simulink model "pipelined_and_spatial_parallelism"  (R2015b)
settings: Solver=FixedStepDiscrete  SolverMode=SingleTasking  StartTime=0.0  StopTime=5e-4  RelTol=1e-3
undefined symbols (not defined in the file): a, b
libraries: shlslibv1 x5277
(part 3 of 23)

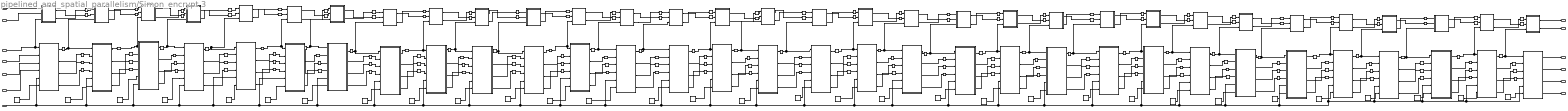
== system pipelined_and_spatial_parallelism/Simon_encrypt 3 ==
  x_i1 : Inport
  x_i : Inport  Port=2
  k_i : Inport  Port=3
  k_i1 : Inport  Port=4
  k_i2 : Inport  Port=5
  k_i3 : Inport  Port=6
  c : Inport  Port=7
  Delay{1..186} (186 alike) : shlslibv1/Memories/Delay  syn_delay_val=1  synBlockType=primitive  synLatency=1  synBlockId=104
  Key_expansion_function : Subsystem
  Key_expansion_function1 : Subsystem
  Key_expansion_function10 : Subsystem
  Key_expansion_function11 : Subsystem
  Key_expansion_function12 : Subsystem
  Key_expansion_function13 : Subsystem
  Key_expansion_function14 : Subsystem
  Key_expansion_function15 : Subsystem
  Key_expansion_function16 : Subsystem
  Key_expansion_function17 : Subsystem
  Key_expansion_function18 : Subsystem
  Key_expansion_function19 : Subsystem
  Key_expansion_function2 : Subsystem
  Key_expansion_function20 : Subsystem
  Key_expansion_function21 : Subsystem
  Key_expansion_function22 : Subsystem
  Key_expansion_function23 : Subsystem
  Key_expansion_function24 : Subsystem
  Key_expansion_function25 : Subsystem
  Key_expansion_function26 : Subsystem
  Key_expansion_function27 : Subsystem
  Key_expansion_function29 : Subsystem
  Key_expansion_function3 : Subsystem
  Key_expansion_function30 : Subsystem
  Key_expansion_function31 : Subsystem
  Key_expansion_function32 : Subsystem
  Key_expansion_function4 : Subsystem
  Key_expansion_function5 : Subsystem
  Key_expansion_function6 : Subsystem
  Key_expansion_function7 : Subsystem
  Key_expansion_function8 : Subsystem
  Key_expansion_function9 : Subsystem
  Round_function : Subsystem
  Round_function1 : Subsystem
  Round_function10 : Subsystem
  Round_function11 : Subsystem
  Round_function12 : Subsystem
  Round_function13 : Subsystem
  Round_function14 : Subsystem
  Round_function15 : Subsystem
  Round_function16 : Subsystem
  Round_function17 : Subsystem
  Round_function18 : Subsystem
  Round_function19 : Subsystem
  Round_function2 : Subsystem
  Round_function20 : Subsystem
  Round_function21 : Subsystem
  Round_function22 : Subsystem
  Round_function23 : Subsystem
  Round_function24 : Subsystem
  Round_function25 : Subsystem
  Round_function26 : Subsystem
  Round_function27 : Subsystem
  Round_function29 : Subsystem
  Round_function3 : Subsystem
  Round_function30 : Subsystem
  Round_function31 : Subsystem
  Round_function32 : Subsystem
  Round_function4 : Subsystem
  Round_function5 : Subsystem
  Round_function6 : Subsystem
  Round_function7 : Subsystem
  Round_function8 : Subsystem
  Round_function9 : Subsystem
  Sequence{,1..4,6,10,13,15,17..18,23..25,28..29} (16 alike) : shlslibv1/Sources/Sequence  syn_seq_vec=[1]  syn_seq_wl=16  syn_seq_fl=0  syn_seq_dt=unsigned  syn_rst_port=off  syn_en_port=off  syn_seq_st=-1  synBlockType=custom  synLatency=1
  Sequence{5,7..9,11..12,14,16,19..22,26..27,30..31} (16 alike) : shlslibv1/Sources/Sequence  syn_seq_vec=[0]  syn_seq_wl=16  syn_seq_fl=0  syn_seq_dt=unsigned  syn_rst_port=off  syn_en_port=off  syn_seq_st=-1  synBlockType=custom  synLatency=1
  X_iiii : Outport
  X_iiii1 : Outport  Port=2
  K_iiii : Outport  Port=3
  K_iiiii1 : Outport  Port=4
  K_iiii2 : Outport  Port=5
  K_iiii3 : Outport  Port=6
  wires:
  Key_expansion_function/2(Kiii1) -> Delay11/1
  Key_expansion_function/3(Kiii2) -> Delay12/1
  Key_expansion_function/4(Kiii3) -> Delay13/1
  x_i1/1 -> Round_function/1(" x_ii1")
  x_i/1 -> Round_function/2(x_ii)
  k_i/1 -> Round_function/3(k_i), Key_expansion_function/1(k_ii)
  k_i1/1 -> Key_expansion_function/2(k_ii1)
  k_i2/1 -> Key_expansion_function/3(k_ii2)
  k_i3/1 -> Key_expansion_function/4(k_ii3)
  Round_function/2(xiii2) -> Delay7/1
  Round_function/1(Xiii1) -> Delay8/1
  Round_function1/1(Xiii1) -> Delay15/1
  Round_function1/2(xiii2) -> Delay14/1
  Key_expansion_function1/2(Kiii1) -> Delay18/1
  Key_expansion_function1/3(Kiii2) -> Delay19/1
  Key_expansion_function1/4(Kiii3) -> Delay20/1
  Round_function2/1(Xiii1) -> Delay22/1
  Round_function2/2(xiii2) -> Delay21/1
  Key_expansion_function2/2(Kiii1) -> Delay25/1
  Key_expansion_function2/3(Kiii2) -> Delay26/1
  Key_expansion_function2/4(Kiii3) -> Delay27/1
  Delay7/1 -> Round_function1/1(" x_ii1")
  Delay8/1 -> Round_function1/2(x_ii)
  Key_expansion_function/1(K_iii) -> Delay9/1
  Delay11/1 -> Key_expansion_function1/2(k_ii1)
  Delay12/1 -> Key_expansion_function1/3(k_ii2)
  Delay13/1 -> Key_expansion_function1/4(k_ii3)
  Delay14/1 -> Round_function2/1(" x_ii1")
  Delay15/1 -> Round_function2/2(x_ii)
  Key_expansion_function1/1(K_iii) -> Delay10/1
  Delay18/1 -> Key_expansion_function2/2(k_ii1)
  Delay19/1 -> Key_expansion_function2/3(k_ii2)
  Delay20/1 -> Key_expansion_function2/4(k_ii3)
  Delay21/1 -> Round_function3/1(" x_ii1")
  Delay22/1 -> Round_function3/2(x_ii)
  Key_expansion_function2/1(K_iii) -> Delay16/1
  Delay25/1 -> Key_expansion_function3/2(k_ii1)
  Delay26/1 -> Key_expansion_function3/3(k_ii2)
  Delay27/1 -> Key_expansion_function3/4(k_ii3)
  Delay9/1 -> Key_expansion_function1/1(k_ii), Round_function1/3(k_i)
  Delay10/1 -> Round_function2/3(k_i), Key_expansion_function2/1(k_ii)
  Delay16/1 -> Key_expansion_function3/1(k_ii), Round_function3/3(k_i)
  Key_expansion_function3/2(Kiii1) -> Delay2/1
  Key_expansion_function3/3(Kiii2) -> Delay3/1
  Key_expansion_function3/4(Kiii3) -> Delay4/1
  Round_function3/2(xiii2) -> Delay34/1
  Round_function3/1(Xiii1) -> Delay35/1
  Round_function4/1(Xiii1) -> Delay6/1
  Round_function4/2(xiii2) -> Delay5/1
  Key_expansion_function4/2(Kiii1) -> Delay23/1
  Key_expansion_function4/3(Kiii2) -> Delay24/1
  Key_expansion_function4/4(Kiii3) -> Delay28/1
  Round_function5/1(Xiii1) -> Delay30/1
  Round_function5/2(xiii2) -> Delay29/1
  Key_expansion_function5/2(Kiii1) -> Delay31/1
  Key_expansion_function5/3(Kiii2) -> Delay32/1
  Key_expansion_function5/4(Kiii3) -> Delay33/1
  Delay34/1 -> Round_function4/1(" x_ii1")
  Delay35/1 -> Round_function4/2(x_ii)
  Key_expansion_function3/1(K_iii) -> Delay36/1
  Delay2/1 -> Key_expansion_function4/2(k_ii1)
  Delay3/1 -> Key_expansion_function4/3(k_ii2)
  Delay4/1 -> Key_expansion_function4/4(k_ii3)
  Delay5/1 -> Round_function5/1(" x_ii1")
  Delay6/1 -> Round_function5/2(x_ii)
  Key_expansion_function4/1(K_iii) -> Delay1/1
  Delay23/1 -> Key_expansion_function5/2(k_ii1)
  Delay24/1 -> Key_expansion_function5/3(k_ii2)
  Delay28/1 -> Key_expansion_function5/4(k_ii3)
  Delay29/1 -> Round_function6/1(" x_ii1")
  Delay30/1 -> Round_function6/2(x_ii)
  Key_expansion_function5/1(K_iii) -> Delay17/1
  Delay31/1 -> Key_expansion_function6/2(k_ii1)
  Delay32/1 -> Key_expansion_function6/3(k_ii2)
  Delay33/1 -> Key_expansion_function6/4(k_ii3)
  Delay36/1 -> Round_function4/3(k_i), Key_expansion_function4/1(k_ii)
  Delay1/1 -> Key_expansion_function5/1(k_ii), Round_function5/3(k_i)
  Delay17/1 -> Key_expansion_function6/1(k_ii), Round_function6/3(k_i)
  Key_expansion_function6/2(Kiii1) -> Delay39/1
  Key_expansion_function6/3(Kiii2) -> Delay40/1
  Key_expansion_function6/4(Kiii3) -> Delay41/1
  Round_function6/2(xiii2) -> Delay70/1
  Round_function6/1(Xiii1) -> Delay71/1
  Round_function7/1(Xiii1) -> Delay43/1
  Round_function7/2(xiii2) -> Delay42/1
  Key_expansion_function7/2(Kiii1) -> Delay46/1
  Key_expansion_function7/3(Kiii2) -> Delay47/1
  Key_expansion_function7/4(Kiii3) -> Delay49/1
  Round_function8/1(Xiii1) -> Delay51/1
  Round_function8/2(xiii2) -> Delay50/1
  Key_expansion_function8/2(Kiii1) -> Delay54/1
  Key_expansion_function8/3(Kiii2) -> Delay55/1
  Key_expansion_function8/4(Kiii3) -> Delay56/1
  Delay70/1 -> Round_function7/1(" x_ii1")
  Delay71/1 -> Round_function7/2(x_ii)
  Key_expansion_function6/1(K_iii) -> Delay72/1
  Delay39/1 -> Key_expansion_function7/2(k_ii1)
  Delay40/1 -> Key_expansion_function7/3(k_ii2)
  Delay41/1 -> Key_expansion_function7/4(k_ii3)
  Delay42/1 -> Round_function8/1(" x_ii1")
  Delay43/1 -> Round_function8/2(x_ii)
  Key_expansion_function7/1(K_iii) -> Delay38/1
  Delay46/1 -> Key_expansion_function8/2(k_ii1)
  Delay47/1 -> Key_expansion_function8/3(k_ii2)
  Delay49/1 -> Key_expansion_function8/4(k_ii3)
  Delay50/1 -> Round_function9/1(" x_ii1")
  Delay51/1 -> Round_function9/2(x_ii)
  Key_expansion_function8/1(K_iii) -> Delay44/1
  Delay54/1 -> Key_expansion_function9/2(k_ii1)
  Delay55/1 -> Key_expansion_function9/3(k_ii2)
  Delay56/1 -> Key_expansion_function9/4(k_ii3)
  Delay72/1 -> Round_function7/3(k_i), Key_expansion_function7/1(k_ii)
  Delay38/1 -> Round_function8/3(k_i), Key_expansion_function8/1(k_ii)
  Delay44/1 -> Round_function9/3(k_i), Key_expansion_function9/1(k_ii)
  Key_expansion_function9/2(Kiii1) -> Delay48/1
  Key_expansion_function9/3(Kiii2) -> Delay59/1
  Key_expansion_function9/4(Kiii3) -> Delay67/1
  Round_function9/2(xiii2) -> Delay64/1
  Round_function9/1(Xiii1) -> Delay65/1
  Round_function10/1(Xiii1) -> Delay69/1
  Round_function10/2(xiii2) -> Delay68/1
  Key_expansion_function10/2(Kiii1) -> Delay52/1
  Key_expansion_function10/3(Kiii2) -> Delay53/1
  Key_expansion_function10/4(Kiii3) -> Delay57/1
  Round_function11/1(Xiii1) -> Delay60/1
  Round_function11/2(xiii2) -> Delay58/1
  Key_expansion_function11/2(Kiii1) -> Delay61/1
  Key_expansion_function11/3(Kiii2) -> Delay62/1
  Key_expansion_function11/4(Kiii3) -> Delay63/1
  Delay64/1 -> Round_function10/1(" x_ii1")
  Delay65/1 -> Round_function10/2(x_ii)
  Key_expansion_function9/1(K_iii) -> Delay66/1
  Delay48/1 -> Key_expansion_function10/2(k_ii1)
  Delay59/1 -> Key_expansion_function10/3(k_ii2)
  Delay67/1 -> Key_expansion_function10/4(k_ii3)
  Delay68/1 -> Round_function11/1(" x_ii1")
  Delay69/1 -> Round_function11/2(x_ii)
  Key_expansion_function10/1(K_iii) -> Delay37/1
  Delay52/1 -> Key_expansion_function11/2(k_ii1)
  Delay53/1 -> Key_expansion_function11/3(k_ii2)
  Delay57/1 -> Key_expansion_function11/4(k_ii3)
  Delay58/1 -> Round_function12/1(" x_ii1")
  Delay60/1 -> Round_function12/2(x_ii)
  Key_expansion_function11/1(K_iii) -> Delay45/1
  Delay61/1 -> Key_expansion_function12/2(k_ii1)
  Delay62/1 -> Key_expansion_function12/3(k_ii2)
  Delay63/1 -> Key_expansion_function12/4(k_ii3)
  Delay66/1 -> Round_function10/3(k_i), Key_expansion_function10/1(k_ii)
  Delay37/1 -> Key_expansion_function11/1(k_ii), Round_function11/3(k_i)
  Delay45/1 -> Round_function12/3(k_i), Key_expansion_function12/1(k_ii)
  Key_expansion_function12/2(Kiii1) -> Delay75/1
  Key_expansion_function12/3(Kiii2) -> Delay76/1
  Key_expansion_function12/4(Kiii3) -> Delay77/1
  Round_function12/2(xiii2) -> Delay139/1
  Round_function12/1(Xiii1) -> Delay143/1
  Round_function13/1(Xiii1) -> Delay79/1
  Round_function13/2(xiii2) -> Delay78/1
  Key_expansion_function13/2(Kiii1) -> Delay82/1
  Key_expansion_function13/3(Kiii2) -> Delay83/1
  Key_expansion_function13/4(Kiii3) -> Delay85/1
  Round_function14/1(Xiii1) -> Delay87/1
  Round_function14/2(xiii2) -> Delay86/1
  Key_expansion_function14/2(Kiii1) -> Delay90/1
  Key_expansion_function14/3(Kiii2) -> Delay91/1
  Key_expansion_function14/4(Kiii3) -> Delay92/1
  Delay139/1 -> Round_function13/1(" x_ii1")
  Delay143/1 -> Round_function13/2(x_ii)
  Key_expansion_function12/1(K_iii) -> Delay144/1
  Delay75/1 -> Key_expansion_function13/2(k_ii1)
  Delay76/1 -> Key_expansion_function13/3(k_ii2)
  Delay77/1 -> Key_expansion_function13/4(k_ii3)
  Delay78/1 -> Round_function14/1(" x_ii1")
  Delay79/1 -> Round_function14/2(x_ii)
  Key_expansion_function13/1(K_iii) -> Delay74/1
  Delay82/1 -> Key_expansion_function14/2(k_ii1)
  Delay83/1 -> Key_expansion_function14/3(k_ii2)
  Delay85/1 -> Key_expansion_function14/4(k_ii3)
  Delay86/1 -> Round_function15/1(" x_ii1")
  Delay87/1 -> Round_function15/2(x_ii)
  Key_expansion_function14/1(K_iii) -> Delay80/1
  Delay90/1 -> Key_expansion_function15/2(k_ii1)
  Delay91/1 -> Key_expansion_function15/3(k_ii2)
  Delay92/1 -> Key_expansion_function15/4(k_ii3)
  Delay144/1 -> Round_function13/3(k_i), Key_expansion_function13/1(k_ii)
  Delay74/1 -> Round_function14/3(k_i), Key_expansion_function14/1(k_ii)
  Delay80/1 -> Round_function15/3(k_i), Key_expansion_function15/1(k_ii)
  Key_expansion_function15/2(Kiii1) -> Delay84/1
  Key_expansion_function15/3(Kiii2) -> Delay95/1
  Key_expansion_function15/4(Kiii3) -> Delay106/1
  Round_function15/2(xiii2) -> Delay100/1
  Round_function15/1(Xiii1) -> Delay101/1
  Round_function16/1(Xiii1) -> Delay128/1
  Round_function16/2(xiii2) -> Delay117/1
  Key_expansion_function16/2(Kiii1) -> Delay88/1
  Key_expansion_function16/3(Kiii2) -> Delay89/1
  Key_expansion_function16/4(Kiii3) -> Delay93/1
  Round_function17/1(Xiii1) -> Delay96/1
  Round_function17/2(xiii2) -> Delay94/1
  Key_expansion_function17/2(Kiii1) -> Delay97/1
  Key_expansion_function17/3(Kiii2) -> Delay98/1
  Key_expansion_function17/4(Kiii3) -> Delay99/1
  Delay100/1 -> Round_function16/1(" x_ii1")
  Delay101/1 -> Round_function16/2(x_ii)
  Key_expansion_function15/1(K_iii) -> Delay102/1
  Delay84/1 -> Key_expansion_function16/2(k_ii1)
  Delay95/1 -> Key_expansion_function16/3(k_ii2)
  Delay106/1 -> Key_expansion_function16/4(k_ii3)
  Delay117/1 -> Round_function17/1(" x_ii1")
  Delay128/1 -> Round_function17/2(x_ii)
  Key_expansion_function16/1(K_iii) -> Delay73/1
  Delay88/1 -> Key_expansion_function17/2(k_ii1)
  Delay89/1 -> Key_expansion_function17/3(k_ii2)
  Delay93/1 -> Key_expansion_function17/4(k_ii3)
  Delay94/1 -> Round_function18/1(" x_ii1")
  Delay96/1 -> Round_function18/2(x_ii)
  Key_expansion_function17/1(K_iii) -> Delay81/1
  Delay97/1 -> Key_expansion_function18/2(k_ii1)
  Delay98/1 -> Key_expansion_function18/3(k_ii2)
  Delay99/1 -> Key_expansion_function18/4(k_ii3)
  Delay102/1 -> Round_function16/3(k_i), Key_expansion_function16/1(k_ii)
  Delay73/1 -> Key_expansion_function17/1(k_ii), Round_function17/3(k_i)
  Delay81/1 -> Key_expansion_function18/1(k_ii), Round_function18/3(k_i)
  Key_expansion_function18/2(Kiii1) -> Delay105/1
  Key_expansion_function18/3(Kiii2) -> Delay107/1
  Key_expansion_function18/4(Kiii3) -> Delay108/1
  Round_function18/2(xiii2) -> Delay140/1
  Round_function18/1(Xiii1) -> Delay141/1
  Round_function19/1(Xiii1) -> Delay110/1
  Round_function19/2(xiii2) -> Delay109/1
  Key_expansion_function19/2(Kiii1) -> Delay113/1
  Key_expansion_function19/3(Kiii2) -> Delay114/1
  Key_expansion_function19/4(Kiii3) -> Delay116/1
  Round_function20/1(Xiii1) -> Delay119/1
  Round_function20/2(xiii2) -> Delay118/1
  Key_expansion_function20/2(Kiii1) -> Delay122/1
  Key_expansion_function20/3(Kiii2) -> Delay123/1
  Key_expansion_function20/4(Kiii3) -> Delay124/1
  Delay140/1 -> Round_function19/1(" x_ii1")
  Delay141/1 -> Round_function19/2(x_ii)
  Key_expansion_function18/1(K_iii) -> Delay142/1
  Delay105/1 -> Key_expansion_function19/2(k_ii1)
  Delay107/1 -> Key_expansion_function19/3(k_ii2)
  Delay108/1 -> Key_expansion_function19/4(k_ii3)
  Delay109/1 -> Round_function20/1(" x_ii1")
  Delay110/1 -> Round_function20/2(x_ii)
  Key_expansion_function19/1(K_iii) -> Delay104/1
  Delay113/1 -> Key_expansion_function20/2(k_ii1)
  Delay114/1 -> Key_expansion_function20/3(k_ii2)
  Delay116/1 -> Key_expansion_function20/4(k_ii3)
  Delay118/1 -> Round_function21/1(" x_ii1")
  Delay119/1 -> Round_function21/2(x_ii)
  Key_expansion_function20/1(K_iii) -> Delay111/1
  Delay122/1 -> Key_expansion_function21/2(k_ii1)
  Delay123/1 -> Key_expansion_function21/3(k_ii2)
  Delay124/1 -> Key_expansion_function21/4(k_ii3)
  Delay142/1 -> Round_function19/3(k_i), Key_expansion_function19/1(k_ii)
  Delay104/1 -> Round_function20/3(k_i), Key_expansion_function20/1(k_ii)
  Delay111/1 -> Key_expansion_function21/1(k_ii), Round_function21/3(k_i)
  Key_expansion_function21/2(Kiii1) -> Delay115/1
  Key_expansion_function21/3(Kiii2) -> Delay127/1
  Key_expansion_function21/4(Kiii3) -> Delay136/1
  Round_function21/2(xiii2) -> Delay133/1
  Round_function21/1(Xiii1) -> Delay134/1
  Round_function22/1(Xiii1) -> Delay138/1
  Round_function22/2(xiii2) -> Delay137/1
  Key_expansion_function22/2(Kiii1) -> Delay120/1
  Key_expansion_function22/3(Kiii2) -> Delay121/1
  Key_expansion_function22/4(Kiii3) -> Delay125/1
  Round_function23/1(Xiii1) -> Delay129/1
  Round_function23/2(xiii2) -> Delay126/1
  Key_expansion_function23/2(Kiii1) -> Delay130/1
  Key_expansion_function23/3(Kiii2) -> Delay131/1
  Key_expansion_function23/4(Kiii3) -> Delay132/1
  Delay133/1 -> Round_function22/1(" x_ii1")
  Delay134/1 -> Round_function22/2(x_ii)
  Key_expansion_function21/1(K_iii) -> Delay135/1
  Delay115/1 -> Key_expansion_function22/2(k_ii1)
  Delay127/1 -> Key_expansion_function22/3(k_ii2)
  Delay136/1 -> Key_expansion_function22/4(k_ii3)
  Delay137/1 -> Round_function23/1(" x_ii1")
  Delay138/1 -> Round_function23/2(x_ii)
  Key_expansion_function22/1(K_iii) -> Delay103/1
  Delay120/1 -> Key_expansion_function23/2(k_ii1)
  Delay121/1 -> Key_expansion_function23/3(k_ii2)
  Delay125/1 -> Key_expansion_function23/4(k_ii3)
  Delay126/1 -> Round_function24/1(" x_ii1")
  Delay129/1 -> Round_function24/2(x_ii)
  Key_expansion_function23/1(K_iii) -> Delay112/1
  Delay130/1 -> Key_expansion_function24/2(k_ii1)
  Delay131/1 -> Key_expansion_function24/3(k_ii2)
  Delay132/1 -> Key_expansion_function24/4(k_ii3)
  Delay135/1 -> Round_function22/3(k_i), Key_expansion_function22/1(k_ii)
  Delay103/1 -> Key_expansion_function23/1(k_ii), Round_function23/3(k_i)
  Delay112/1 -> Round_function24/3(k_i), Key_expansion_function24/1(k_ii)
  Round_function24/1(Xiii1) -> Delay183/1
  Round_function24/2(xiii2) -> Delay182/1
  Key_expansion_function24/2(Kiii1) -> Delay184/1
  Key_expansion_function24/3(Kiii2) -> Delay185/1
  Key_expansion_function24/4(Kiii3) -> Delay186/1
  Delay182/1 -> Round_function25/1(" x_ii1")
  Delay183/1 -> Round_function25/2(x_ii)
  Key_expansion_function24/1(K_iii) -> Delay181/1
  Delay184/1 -> Key_expansion_function25/2(k_ii1)
  Delay185/1 -> Key_expansion_function25/3(k_ii2)
  Delay186/1 -> Key_expansion_function25/4(k_ii3)
  Delay181/1 -> Key_expansion_function25/1(k_ii), Round_function25/3(k_i)
  Key_expansion_function25/2(Kiii1) -> Delay147/1
  Key_expansion_function25/3(Kiii2) -> Delay148/1
  Key_expansion_function25/4(Kiii3) -> Delay149/1
  Sequence27/1 -> Key_expansion_function27/6(z)
  Sequence28/1 -> Key_expansion_function29/6(z)
  Round_function25/2(xiii2) -> Delay178/1
  Round_function25/1(Xiii1) -> Delay179/1
  Round_function26/1(Xiii1) -> Delay151/1
  Round_function26/2(xiii2) -> Delay150/1
  Key_expansion_function26/2(Kiii1) -> Delay154/1
  Key_expansion_function26/3(Kiii2) -> Delay155/1
  Key_expansion_function26/4(Kiii3) -> Delay157/1
  Round_function27/1(Xiii1) -> Delay159/1
  Round_function27/2(xiii2) -> Delay158/1
  Key_expansion_function27/2(Kiii1) -> Delay162/1
  Key_expansion_function27/3(Kiii2) -> Delay163/1
  Key_expansion_function27/4(Kiii3) -> Delay164/1
  Delay178/1 -> Round_function26/1(" x_ii1")
  Delay179/1 -> Round_function26/2(x_ii)
  Key_expansion_function25/1(K_iii) -> Delay180/1
  Delay147/1 -> Key_expansion_function26/2(k_ii1)
  Delay148/1 -> Key_expansion_function26/3(k_ii2)
  Delay149/1 -> Key_expansion_function26/4(k_ii3)
  Delay150/1 -> Round_function27/1(" x_ii1")
  Delay151/1 -> Round_function27/2(x_ii)
  Key_expansion_function26/1(K_iii) -> Delay146/1
  Delay154/1 -> Key_expansion_function27/2(k_ii1)
  Delay155/1 -> Key_expansion_function27/3(k_ii2)
  Delay157/1 -> Key_expansion_function27/4(k_ii3)
  Delay158/1 -> Round_function29/1(" x_ii1")
  Delay159/1 -> Round_function29/2(x_ii)
  Key_expansion_function27/1(K_iii) -> Delay152/1
  Delay162/1 -> Key_expansion_function29/2(k_ii1)
  Delay163/1 -> Key_expansion_function29/3(k_ii2)
  Delay164/1 -> Key_expansion_function29/4(k_ii3)
  Delay180/1 -> Round_function26/3(k_i), Key_expansion_function26/1(k_ii)
  Delay146/1 -> Round_function27/3(k_i), Key_expansion_function27/1(k_ii)
  Delay152/1 -> Round_function29/3(k_i), Key_expansion_function29/1(k_ii)
  Key_expansion_function29/2(Kiii1) -> Delay156/1
  Key_expansion_function29/3(Kiii2) -> Delay167/1
  Key_expansion_function29/4(Kiii3) -> Delay175/1
  Sequence30/1 -> Key_expansion_function31/6(z)
  Round_function29/2(xiii2) -> Delay172/1
  Round_function29/1(Xiii1) -> Delay173/1
  Round_function30/1(Xiii1) -> Delay177/1
  Round_function30/2(xiii2) -> Delay176/1
  Key_expansion_function30/2(Kiii1) -> Delay160/1
  Key_expansion_function30/3(Kiii2) -> Delay161/1
  Key_expansion_function30/4(Kiii3) -> Delay165/1
  Round_function31/1(Xiii1) -> Delay168/1
  Round_function31/2(xiii2) -> Delay166/1
  Key_expansion_function31/2(Kiii1) -> Delay169/1
  Key_expansion_function31/3(Kiii2) -> Delay170/1
  Key_expansion_function31/4(Kiii3) -> Delay171/1
  Delay172/1 -> Round_function30/1(" x_ii1")
  Delay173/1 -> Round_function30/2(x_ii)
  Key_expansion_function29/1(K_iii) -> Delay174/1
  Delay156/1 -> Key_expansion_function30/2(k_ii1)
  Delay167/1 -> Key_expansion_function30/3(k_ii2)
  Delay175/1 -> Key_expansion_function30/4(k_ii3)
  Delay176/1 -> Round_function31/1(" x_ii1")
  Delay177/1 -> Round_function31/2(x_ii)
  Key_expansion_function30/1(K_iii) -> Delay145/1
  Delay160/1 -> Key_expansion_function31/2(k_ii1)
  Delay161/1 -> Key_expansion_function31/3(k_ii2)
  Delay165/1 -> Key_expansion_function31/4(k_ii3)
  Delay166/1 -> Round_function32/1(" x_ii1")
  Delay168/1 -> Round_function32/2(x_ii)
  Key_expansion_function31/1(K_iii) -> Delay153/1
  Delay169/1 -> Key_expansion_function32/2(k_ii1)
  Delay170/1 -> Key_expansion_function32/3(k_ii2)
  Delay171/1 -> Key_expansion_function32/4(k_ii3)
  Delay174/1 -> Round_function30/3(k_i), Key_expansion_function30/1(k_ii)
  Delay145/1 -> Round_function31/3(k_i), Key_expansion_function31/1(k_ii)
  Delay153/1 -> Key_expansion_function32/1(k_ii), Round_function32/3(k_i)
  c/1 -> Key_expansion_function1/5(c), Key_expansion_function2/6(z), Key_expansion_function3/6(z), Key_expansion_function4/5(c), Key_expansion_function5/5(c), Key_expansion_function6/5(c), Key_expansion_function7/5(c), Key_expansion_function8/5(c), Key_expansion_function9/5(c), Key_expansion_function10/5(c), Key_expansion_function11/5(c), Key_expansion_function12/5(c), Key_expansion_function13/5(c), Key_expansion_function14/5(c), Key_expansion_function15/5(c), Key_expansion_function16/5(c), Key_expansion_function17/5(c), Key_expansion_function18/5(c), Key_expansion_function19/5(c), Key_expansion_function20/5(c), Key_expansion_function21/5(c), Key_expansion_function22/5(c), Key_expansion_function23/5(c), Key_expansion_function24/5(c), Key_expansion_function25/5(c), Key_expansion_function26/5(c), Key_expansion_function27/5(c), Key_expansion_function29/5(c), Key_expansion_function30/5(c), Key_expansion_function32/5(c), Key_expansion_function31/5(c), Key_expansion_function/5(c)
  Sequence/1 -> Key_expansion_function/6(z)
  Sequence1/1 -> Key_expansion_function1/6(z)
  Sequence2/1 -> Key_expansion_function2/5(c)
  Sequence3/1 -> Key_expansion_function3/5(c)
  Sequence4/1 -> Key_expansion_function4/6(z)
  Sequence5/1 -> Key_expansion_function5/6(z)
  Sequence6/1 -> Key_expansion_function6/6(z)
  Sequence7/1 -> Key_expansion_function7/6(z)
  Sequence8/1 -> Key_expansion_function8/6(z)
  Sequence9/1 -> Key_expansion_function9/6(z)
  Sequence10/1 -> Key_expansion_function10/6(z)
  Sequence11/1 -> Key_expansion_function11/6(z)
  Sequence12/1 -> Key_expansion_function12/6(z)
  Sequence13/1 -> Key_expansion_function13/6(z)
  Sequence14/1 -> Key_expansion_function14/6(z)
  Sequence15/1 -> Key_expansion_function15/6(z)
  Sequence16/1 -> Key_expansion_function16/6(z)
  Sequence17/1 -> Key_expansion_function17/6(z)
  Sequence18/1 -> Key_expansion_function18/6(z)
  Sequence19/1 -> Key_expansion_function19/6(z)
  Sequence20/1 -> Key_expansion_function20/6(z)
  Sequence21/1 -> Key_expansion_function21/6(z)
  Sequence22/1 -> Key_expansion_function22/6(z)
  Sequence23/1 -> Key_expansion_function23/6(z)
  Sequence29/1 -> Key_expansion_function30/6(z)
  Sequence26/1 -> Key_expansion_function26/6(z)
  Sequence31/1 -> Key_expansion_function32/6(z)
  Sequence25/1 -> Key_expansion_function25/6(z)
  Sequence24/1 -> Key_expansion_function24/6(z)
  Round_function32/1(Xiii1) -> X_iiii/1
  Round_function32/2(xiii2) -> X_iiii1/1
  Key_expansion_function32/1(K_iii) -> K_iiii/1
  Key_expansion_function32/2(Kiii1) -> K_iiiii1/1
  Key_expansion_function32/3(Kiii2) -> K_iiii2/1
  Key_expansion_function32/4(Kiii3) -> K_iiii3/1

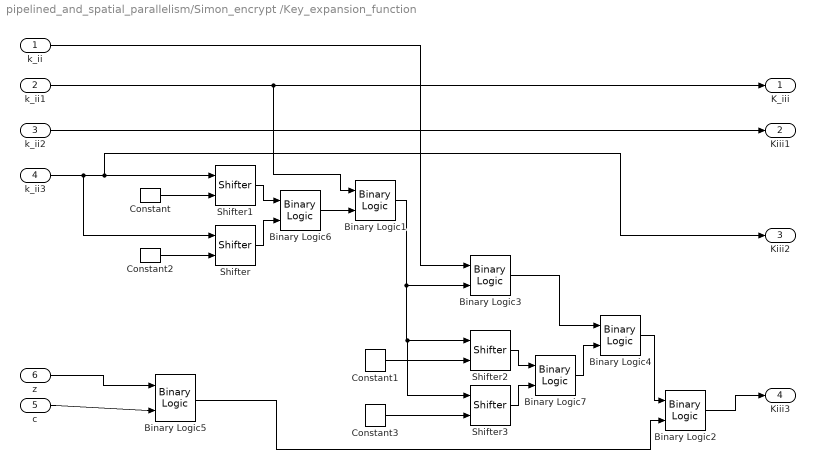
== system pipelined_and_spatial_parallelism/Simon_encrypt /Key_expansion_function ==
  k_ii : Inport
  k_ii1 : Inport  Port=2
  k_ii2 : Inport  Port=3
  k_ii3 : Inport  Port=4
  c : Inport  Port=5
  z : Inport  Port=6
  Binary Logic{1..5} (5 alike) : shlslibv1/Math Functions/Binary Logic  syn_binlog_exp=a^b  synBlockType=primitive  synLatency=0  synBlockId=13
  Binary Logic6 : shlslibv1/Math Functions/Binary Logic  syn_binlog_exp=a|b  synBlockType=primitive  synLatency=0  synBlockId=13
  Binary Logic7 : shlslibv1/Math Functions/Binary Logic  syn_binlog_exp=a|b  synBlockType=primitive  synLatency=0  synBlockId=13
  Constant : shlslibv1/Sources/Constant  syn_cst_val=3  syn_cst_format=Specify  syn_cst_wl=4  syn_cst_fl=0  syn_cst_dt=unsigned  syn_cst_rnd=on  syn_cst_st=-1  synBlockType=primitive  synLatency=0  synBlockId=15
  Constant1 : shlslibv1/Sources/Constant  syn_cst_val=1  syn_cst_format=Specify  syn_cst_wl=4  syn_cst_fl=0  syn_cst_dt=unsigned  syn_cst_rnd=on  syn_cst_st=-1  synBlockType=primitive  synLatency=0  synBlockId=15
  Constant2 : shlslibv1/Sources/Constant  syn_cst_val=13  syn_cst_format=Specify  syn_cst_wl=4  syn_cst_fl=0  syn_cst_dt=unsigned  syn_cst_rnd=on  syn_cst_st=-1  synBlockType=primitive  synLatency=0  synBlockId=15
  Constant3 : shlslibv1/Sources/Constant  syn_cst_val=15  syn_cst_format=Specify  syn_cst_wl=4  syn_cst_fl=0  syn_cst_dt=unsigned  syn_cst_rnd=on  syn_cst_st=-1  synBlockType=primitive  synLatency=0  synBlockId=15
  Shifter : shlslibv1/Math Functions/Shifter  syn_shifter_opr=<<  syn_out_f=Automatic  syn_out_wl=16  syn_out_fl=8  syn_out_dt=signed  synBlockType=primitive  synLatency=0  synBlockId=12
  Shifter1 : shlslibv1/Math Functions/Shifter  syn_shifter_opr=>>  syn_out_f=Automatic  syn_out_wl=16  syn_out_fl=8  syn_out_dt=signed  synBlockType=primitive  synLatency=0  synBlockId=12
  Shifter2 : shlslibv1/Math Functions/Shifter  syn_shifter_opr=>>  syn_out_f=Automatic  syn_out_wl=16  syn_out_fl=8  syn_out_dt=signed  synBlockType=primitive  synLatency=0  synBlockId=12
  Shifter3 : shlslibv1/Math Functions/Shifter  syn_shifter_opr=<<  syn_out_f=Automatic  syn_out_wl=16  syn_out_fl=8  syn_out_dt=signed  synBlockType=primitive  synLatency=0  synBlockId=12
  K_iii : Outport
  Kiii1 : Outport  Port=2
  Kiii2 : Outport  Port=3
  Kiii3 : Outport  Port=4
  wires:
  Binary Logic1/1 -> Shifter3/1, Shifter2/1, Binary Logic3/2
  Constant/1 -> Shifter1/2
  Constant1/1 -> Shifter2/2
  Binary Logic2/1 -> Kiii3/1
  Binary Logic4/1 -> Binary Logic2/1
  k_ii/1 -> Binary Logic3/1
  k_ii1/1 -> K_iii/1, Binary Logic1/1
  z/1 -> Binary Logic5/1
  c/1 -> Binary Logic5/2
  k_ii2/1 -> Kiii1/1
  k_ii3/1 -> Shifter/1, Shifter1/1, Kiii2/1
  Binary Logic3/1 -> Binary Logic4/1
  Binary Logic5/1 -> Binary Logic2/2
  Constant2/1 -> Shifter/2
  Shifter1/1 -> Binary Logic6/1
  Shifter/1 -> Binary Logic6/2
  Binary Logic6/1 -> Binary Logic1/2
  Constant3/1 -> Shifter3/2
  Shifter2/1 -> Binary Logic7/1
  Shifter3/1 -> Binary Logic7/2
  Binary Logic7/1 -> Binary Logic4/2

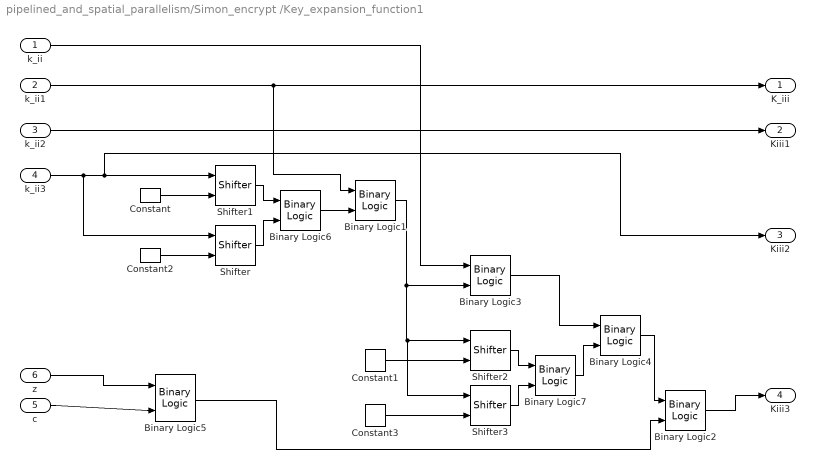
== system pipelined_and_spatial_parallelism/Simon_encrypt /Key_expansion_function1 ==
  k_ii : Inport
  k_ii1 : Inport  Port=2
  k_ii2 : Inport  Port=3
  k_ii3 : Inport  Port=4
  c : Inport  Port=5
  z : Inport  Port=6
  Binary Logic{1..5} (5 alike) : shlslibv1/Math Functions/Binary Logic  syn_binlog_exp=a^b  synBlockType=primitive  synLatency=0  synBlockId=13
  Binary Logic6 : shlslibv1/Math Functions/Binary Logic  syn_binlog_exp=a|b  synBlockType=primitive  synLatency=0  synBlockId=13
  Binary Logic7 : shlslibv1/Math Functions/Binary Logic  syn_binlog_exp=a|b  synBlockType=primitive  synLatency=0  synBlockId=13
  Constant : shlslibv1/Sources/Constant  syn_cst_val=3  syn_cst_format=Specify  syn_cst_wl=4  syn_cst_fl=0  syn_cst_dt=unsigned  syn_cst_rnd=on  syn_cst_st=-1  synBlockType=primitive  synLatency=0  synBlockId=15
  Constant1 : shlslibv1/Sources/Constant  syn_cst_val=1  syn_cst_format=Specify  syn_cst_wl=4  syn_cst_fl=0  syn_cst_dt=unsigned  syn_cst_rnd=on  syn_cst_st=-1  synBlockType=primitive  synLatency=0  synBlockId=15
  Constant2 : shlslibv1/Sources/Constant  syn_cst_val=13  syn_cst_format=Specify  syn_cst_wl=4  syn_cst_fl=0  syn_cst_dt=unsigned  syn_cst_rnd=on  syn_cst_st=-1  synBlockType=primitive  synLatency=0  synBlockId=15
  Constant3 : shlslibv1/Sources/Constant  syn_cst_val=15  syn_cst_format=Specify  syn_cst_wl=4  syn_cst_fl=0  syn_cst_dt=unsigned  syn_cst_rnd=on  syn_cst_st=-1  synBlockType=primitive  synLatency=0  synBlockId=15
  Shifter : shlslibv1/Math Functions/Shifter  syn_shifter_opr=<<  syn_out_f=Automatic  syn_out_wl=16  syn_out_fl=8  syn_out_dt=signed  synBlockType=primitive  synLatency=0  synBlockId=12
  Shifter1 : shlslibv1/Math Functions/Shifter  syn_shifter_opr=>>  syn_out_f=Automatic  syn_out_wl=16  syn_out_fl=8  syn_out_dt=signed  synBlockType=primitive  synLatency=0  synBlockId=12
  Shifter2 : shlslibv1/Math Functions/Shifter  syn_shifter_opr=>>  syn_out_f=Automatic  syn_out_wl=16  syn_out_fl=8  syn_out_dt=signed  synBlockType=primitive  synLatency=0  synBlockId=12
  Shifter3 : shlslibv1/Math Functions/Shifter  syn_shifter_opr=<<  syn_out_f=Automatic  syn_out_wl=16  syn_out_fl=8  syn_out_dt=signed  synBlockType=primitive  synLatency=0  synBlockId=12
  K_iii : Outport
  Kiii1 : Outport  Port=2
  Kiii2 : Outport  Port=3
  Kiii3 : Outport  Port=4
  wires:
  Binary Logic1/1 -> Shifter3/1, Shifter2/1, Binary Logic3/2
  Constant/1 -> Shifter1/2
  Constant1/1 -> Shifter2/2
  Binary Logic2/1 -> Kiii3/1
  Binary Logic4/1 -> Binary Logic2/1
  k_ii/1 -> Binary Logic3/1
  k_ii1/1 -> K_iii/1, Binary Logic1/1
  z/1 -> Binary Logic5/1
  c/1 -> Binary Logic5/2
  k_ii2/1 -> Kiii1/1
  k_ii3/1 -> Shifter/1, Shifter1/1, Kiii2/1
  Binary Logic3/1 -> Binary Logic4/1
  Binary Logic5/1 -> Binary Logic2/2
  Constant2/1 -> Shifter/2
  Shifter1/1 -> Binary Logic6/1
  Shifter/1 -> Binary Logic6/2
  Binary Logic6/1 -> Binary Logic1/2
  Constant3/1 -> Shifter3/2
  Shifter2/1 -> Binary Logic7/1
  Shifter3/1 -> Binary Logic7/2
  Binary Logic7/1 -> Binary Logic4/2

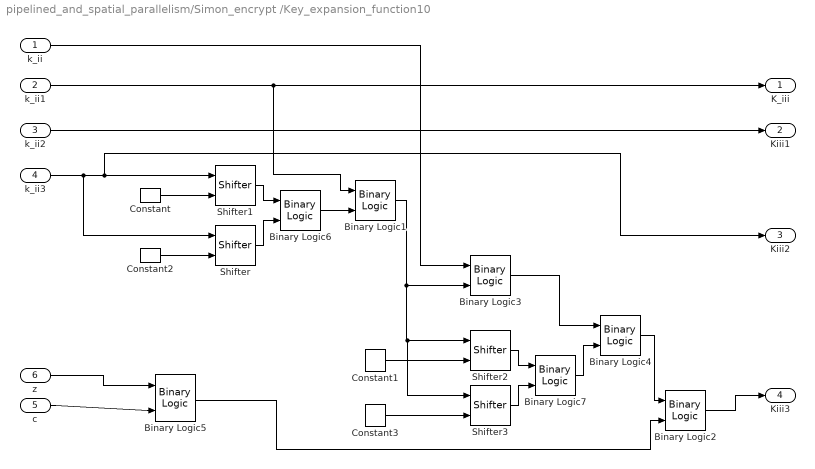
== system pipelined_and_spatial_parallelism/Simon_encrypt /Key_expansion_function10 ==
  k_ii : Inport
  k_ii1 : Inport  Port=2
  k_ii2 : Inport  Port=3
  k_ii3 : Inport  Port=4
  c : Inport  Port=5
  z : Inport  Port=6
  Binary Logic{1..5} (5 alike) : shlslibv1/Math Functions/Binary Logic  syn_binlog_exp=a^b  synBlockType=primitive  synLatency=0  synBlockId=13
  Binary Logic6 : shlslibv1/Math Functions/Binary Logic  syn_binlog_exp=a|b  synBlockType=primitive  synLatency=0  synBlockId=13
  Binary Logic7 : shlslibv1/Math Functions/Binary Logic  syn_binlog_exp=a|b  synBlockType=primitive  synLatency=0  synBlockId=13
  Constant : shlslibv1/Sources/Constant  syn_cst_val=3  syn_cst_format=Specify  syn_cst_wl=4  syn_cst_fl=0  syn_cst_dt=unsigned  syn_cst_rnd=on  syn_cst_st=-1  synBlockType=primitive  synLatency=0  synBlockId=15
  Constant1 : shlslibv1/Sources/Constant  syn_cst_val=1  syn_cst_format=Specify  syn_cst_wl=4  syn_cst_fl=0  syn_cst_dt=unsigned  syn_cst_rnd=on  syn_cst_st=-1  synBlockType=primitive  synLatency=0  synBlockId=15
  Constant2 : shlslibv1/Sources/Constant  syn_cst_val=13  syn_cst_format=Specify  syn_cst_wl=4  syn_cst_fl=0  syn_cst_dt=unsigned  syn_cst_rnd=on  syn_cst_st=-1  synBlockType=primitive  synLatency=0  synBlockId=15
  Constant3 : shlslibv1/Sources/Constant  syn_cst_val=15  syn_cst_format=Specify  syn_cst_wl=4  syn_cst_fl=0  syn_cst_dt=unsigned  syn_cst_rnd=on  syn_cst_st=-1  synBlockType=primitive  synLatency=0  synBlockId=15
  Shifter : shlslibv1/Math Functions/Shifter  syn_shifter_opr=<<  syn_out_f=Automatic  syn_out_wl=16  syn_out_fl=8  syn_out_dt=signed  synBlockType=primitive  synLatency=0  synBlockId=12
  Shifter1 : shlslibv1/Math Functions/Shifter  syn_shifter_opr=>>  syn_out_f=Automatic  syn_out_wl=16  syn_out_fl=8  syn_out_dt=signed  synBlockType=primitive  synLatency=0  synBlockId=12
  Shifter2 : shlslibv1/Math Functions/Shifter  syn_shifter_opr=>>  syn_out_f=Automatic  syn_out_wl=16  syn_out_fl=8  syn_out_dt=signed  synBlockType=primitive  synLatency=0  synBlockId=12
  Shifter3 : shlslibv1/Math Functions/Shifter  syn_shifter_opr=<<  syn_out_f=Automatic  syn_out_wl=16  syn_out_fl=8  syn_out_dt=signed  synBlockType=primitive  synLatency=0  synBlockId=12
  K_iii : Outport
  Kiii1 : Outport  Port=2
  Kiii2 : Outport  Port=3
  Kiii3 : Outport  Port=4
  wires:
  Binary Logic1/1 -> Shifter3/1, Shifter2/1, Binary Logic3/2
  Constant/1 -> Shifter1/2
  Constant1/1 -> Shifter2/2
  Binary Logic2/1 -> Kiii3/1
  Binary Logic4/1 -> Binary Logic2/1
  k_ii/1 -> Binary Logic3/1
  k_ii1/1 -> K_iii/1, Binary Logic1/1
  z/1 -> Binary Logic5/1
  c/1 -> Binary Logic5/2
  k_ii2/1 -> Kiii1/1
  k_ii3/1 -> Shifter/1, Shifter1/1, Kiii2/1
  Binary Logic3/1 -> Binary Logic4/1
  Binary Logic5/1 -> Binary Logic2/2
  Constant2/1 -> Shifter/2
  Shifter1/1 -> Binary Logic6/1
  Shifter/1 -> Binary Logic6/2
  Binary Logic6/1 -> Binary Logic1/2
  Constant3/1 -> Shifter3/2
  Shifter2/1 -> Binary Logic7/1
  Shifter3/1 -> Binary Logic7/2
  Binary Logic7/1 -> Binary Logic4/2

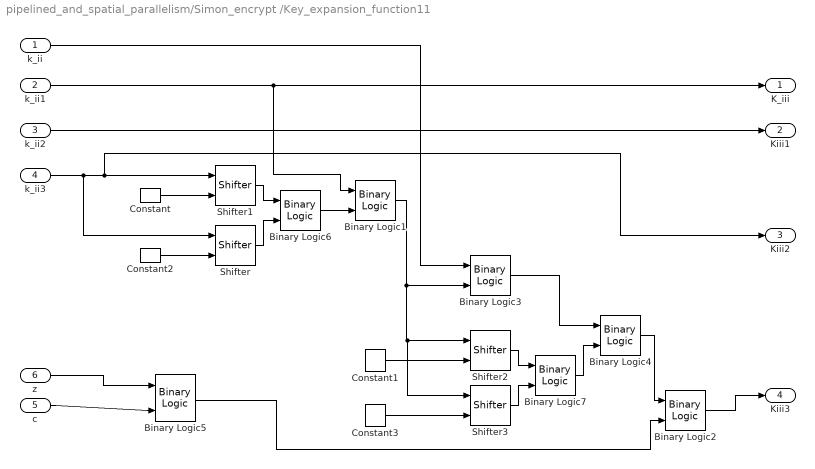
== system pipelined_and_spatial_parallelism/Simon_encrypt /Key_expansion_function11 ==
  k_ii : Inport
  k_ii1 : Inport  Port=2
  k_ii2 : Inport  Port=3
  k_ii3 : Inport  Port=4
  c : Inport  Port=5
  z : Inport  Port=6
  Binary Logic{1..5} (5 alike) : shlslibv1/Math Functions/Binary Logic  syn_binlog_exp=a^b  synBlockType=primitive  synLatency=0  synBlockId=13
  Binary Logic6 : shlslibv1/Math Functions/Binary Logic  syn_binlog_exp=a|b  synBlockType=primitive  synLatency=0  synBlockId=13
  Binary Logic7 : shlslibv1/Math Functions/Binary Logic  syn_binlog_exp=a|b  synBlockType=primitive  synLatency=0  synBlockId=13
  Constant : shlslibv1/Sources/Constant  syn_cst_val=3  syn_cst_format=Specify  syn_cst_wl=4  syn_cst_fl=0  syn_cst_dt=unsigned  syn_cst_rnd=on  syn_cst_st=-1  synBlockType=primitive  synLatency=0  synBlockId=15
  Constant1 : shlslibv1/Sources/Constant  syn_cst_val=1  syn_cst_format=Specify  syn_cst_wl=4  syn_cst_fl=0  syn_cst_dt=unsigned  syn_cst_rnd=on  syn_cst_st=-1  synBlockType=primitive  synLatency=0  synBlockId=15
  Constant2 : shlslibv1/Sources/Constant  syn_cst_val=13  syn_cst_format=Specify  syn_cst_wl=4  syn_cst_fl=0  syn_cst_dt=unsigned  syn_cst_rnd=on  syn_cst_st=-1  synBlockType=primitive  synLatency=0  synBlockId=15
  Constant3 : shlslibv1/Sources/Constant  syn_cst_val=15  syn_cst_format=Specify  syn_cst_wl=4  syn_cst_fl=0  syn_cst_dt=unsigned  syn_cst_rnd=on  syn_cst_st=-1  synBlockType=primitive  synLatency=0  synBlockId=15
  Shifter : shlslibv1/Math Functions/Shifter  syn_shifter_opr=<<  syn_out_f=Automatic  syn_out_wl=16  syn_out_fl=8  syn_out_dt=signed  synBlockType=primitive  synLatency=0  synBlockId=12
  Shifter1 : shlslibv1/Math Functions/Shifter  syn_shifter_opr=>>  syn_out_f=Automatic  syn_out_wl=16  syn_out_fl=8  syn_out_dt=signed  synBlockType=primitive  synLatency=0  synBlockId=12
  Shifter2 : shlslibv1/Math Functions/Shifter  syn_shifter_opr=>>  syn_out_f=Automatic  syn_out_wl=16  syn_out_fl=8  syn_out_dt=signed  synBlockType=primitive  synLatency=0  synBlockId=12
  Shifter3 : shlslibv1/Math Functions/Shifter  syn_shifter_opr=<<  syn_out_f=Automatic  syn_out_wl=16  syn_out_fl=8  syn_out_dt=signed  synBlockType=primitive  synLatency=0  synBlockId=12
  K_iii : Outport
  Kiii1 : Outport  Port=2
  Kiii2 : Outport  Port=3
  Kiii3 : Outport  Port=4
  wires:
  Binary Logic1/1 -> Shifter3/1, Shifter2/1, Binary Logic3/2
  Constant/1 -> Shifter1/2
  Constant1/1 -> Shifter2/2
  Binary Logic2/1 -> Kiii3/1
  Binary Logic4/1 -> Binary Logic2/1
  k_ii/1 -> Binary Logic3/1
  k_ii1/1 -> K_iii/1, Binary Logic1/1
  z/1 -> Binary Logic5/1
  c/1 -> Binary Logic5/2
  k_ii2/1 -> Kiii1/1
  k_ii3/1 -> Shifter/1, Shifter1/1, Kiii2/1
  Binary Logic3/1 -> Binary Logic4/1
  Binary Logic5/1 -> Binary Logic2/2
  Constant2/1 -> Shifter/2
  Shifter1/1 -> Binary Logic6/1
  Shifter/1 -> Binary Logic6/2
  Binary Logic6/1 -> Binary Logic1/2
  Constant3/1 -> Shifter3/2
  Shifter2/1 -> Binary Logic7/1
  Shifter3/1 -> Binary Logic7/2
  Binary Logic7/1 -> Binary Logic4/2

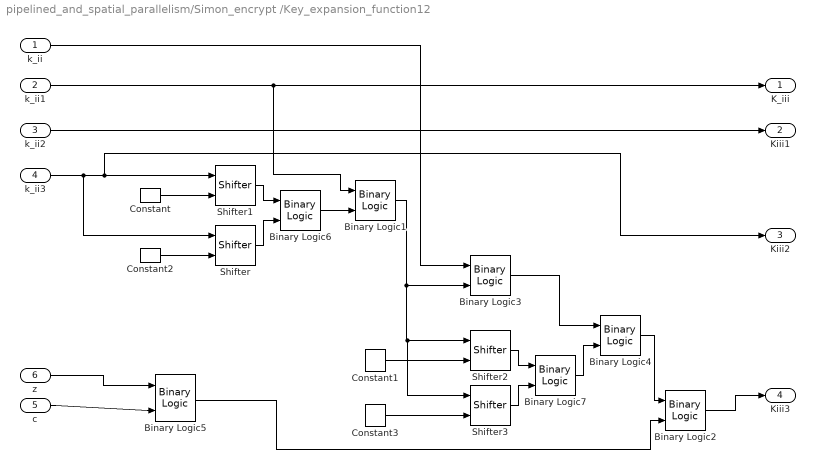
== system pipelined_and_spatial_parallelism/Simon_encrypt /Key_expansion_function12 ==
  k_ii : Inport
  k_ii1 : Inport  Port=2
  k_ii2 : Inport  Port=3
  k_ii3 : Inport  Port=4
  c : Inport  Port=5
  z : Inport  Port=6
  Binary Logic{1..5} (5 alike) : shlslibv1/Math Functions/Binary Logic  syn_binlog_exp=a^b  synBlockType=primitive  synLatency=0  synBlockId=13
  Binary Logic6 : shlslibv1/Math Functions/Binary Logic  syn_binlog_exp=a|b  synBlockType=primitive  synLatency=0  synBlockId=13
  Binary Logic7 : shlslibv1/Math Functions/Binary Logic  syn_binlog_exp=a|b  synBlockType=primitive  synLatency=0  synBlockId=13
  Constant : shlslibv1/Sources/Constant  syn_cst_val=3  syn_cst_format=Specify  syn_cst_wl=4  syn_cst_fl=0  syn_cst_dt=unsigned  syn_cst_rnd=on  syn_cst_st=-1  synBlockType=primitive  synLatency=0  synBlockId=15
  Constant1 : shlslibv1/Sources/Constant  syn_cst_val=1  syn_cst_format=Specify  syn_cst_wl=4  syn_cst_fl=0  syn_cst_dt=unsigned  syn_cst_rnd=on  syn_cst_st=-1  synBlockType=primitive  synLatency=0  synBlockId=15
  Constant2 : shlslibv1/Sources/Constant  syn_cst_val=13  syn_cst_format=Specify  syn_cst_wl=4  syn_cst_fl=0  syn_cst_dt=unsigned  syn_cst_rnd=on  syn_cst_st=-1  synBlockType=primitive  synLatency=0  synBlockId=15
  Constant3 : shlslibv1/Sources/Constant  syn_cst_val=15  syn_cst_format=Specify  syn_cst_wl=4  syn_cst_fl=0  syn_cst_dt=unsigned  syn_cst_rnd=on  syn_cst_st=-1  synBlockType=primitive  synLatency=0  synBlockId=15
  Shifter : shlslibv1/Math Functions/Shifter  syn_shifter_opr=<<  syn_out_f=Automatic  syn_out_wl=16  syn_out_fl=8  syn_out_dt=signed  synBlockType=primitive  synLatency=0  synBlockId=12
  Shifter1 : shlslibv1/Math Functions/Shifter  syn_shifter_opr=>>  syn_out_f=Automatic  syn_out_wl=16  syn_out_fl=8  syn_out_dt=signed  synBlockType=primitive  synLatency=0  synBlockId=12
  Shifter2 : shlslibv1/Math Functions/Shifter  syn_shifter_opr=>>  syn_out_f=Automatic  syn_out_wl=16  syn_out_fl=8  syn_out_dt=signed  synBlockType=primitive  synLatency=0  synBlockId=12
  Shifter3 : shlslibv1/Math Functions/Shifter  syn_shifter_opr=<<  syn_out_f=Automatic  syn_out_wl=16  syn_out_fl=8  syn_out_dt=signed  synBlockType=primitive  synLatency=0  synBlockId=12
  K_iii : Outport
  Kiii1 : Outport  Port=2
  Kiii2 : Outport  Port=3
  Kiii3 : Outport  Port=4
  wires:
  Binary Logic1/1 -> Shifter3/1, Shifter2/1, Binary Logic3/2
  Constant/1 -> Shifter1/2
  Constant1/1 -> Shifter2/2
  Binary Logic2/1 -> Kiii3/1
  Binary Logic4/1 -> Binary Logic2/1
  k_ii/1 -> Binary Logic3/1
  k_ii1/1 -> K_iii/1, Binary Logic1/1
  z/1 -> Binary Logic5/1
  c/1 -> Binary Logic5/2
  k_ii2/1 -> Kiii1/1
  k_ii3/1 -> Shifter/1, Shifter1/1, Kiii2/1
  Binary Logic3/1 -> Binary Logic4/1
  Binary Logic5/1 -> Binary Logic2/2
  Constant2/1 -> Shifter/2
  Shifter1/1 -> Binary Logic6/1
  Shifter/1 -> Binary Logic6/2
  Binary Logic6/1 -> Binary Logic1/2
  Constant3/1 -> Shifter3/2
  Shifter2/1 -> Binary Logic7/1
  Shifter3/1 -> Binary Logic7/2
  Binary Logic7/1 -> Binary Logic4/2

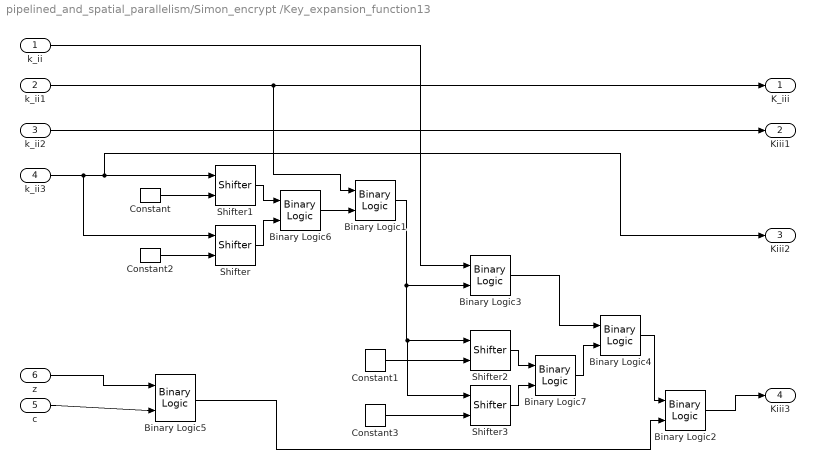
== system pipelined_and_spatial_parallelism/Simon_encrypt /Key_expansion_function13 ==
  k_ii : Inport
  k_ii1 : Inport  Port=2
  k_ii2 : Inport  Port=3
  k_ii3 : Inport  Port=4
  c : Inport  Port=5
  z : Inport  Port=6
  Binary Logic{1..5} (5 alike) : shlslibv1/Math Functions/Binary Logic  syn_binlog_exp=a^b  synBlockType=primitive  synLatency=0  synBlockId=13
  Binary Logic6 : shlslibv1/Math Functions/Binary Logic  syn_binlog_exp=a|b  synBlockType=primitive  synLatency=0  synBlockId=13
  Binary Logic7 : shlslibv1/Math Functions/Binary Logic  syn_binlog_exp=a|b  synBlockType=primitive  synLatency=0  synBlockId=13
  Constant : shlslibv1/Sources/Constant  syn_cst_val=3  syn_cst_format=Specify  syn_cst_wl=4  syn_cst_fl=0  syn_cst_dt=unsigned  syn_cst_rnd=on  syn_cst_st=-1  synBlockType=primitive  synLatency=0  synBlockId=15
  Constant1 : shlslibv1/Sources/Constant  syn_cst_val=1  syn_cst_format=Specify  syn_cst_wl=4  syn_cst_fl=0  syn_cst_dt=unsigned  syn_cst_rnd=on  syn_cst_st=-1  synBlockType=primitive  synLatency=0  synBlockId=15
  Constant2 : shlslibv1/Sources/Constant  syn_cst_val=13  syn_cst_format=Specify  syn_cst_wl=4  syn_cst_fl=0  syn_cst_dt=unsigned  syn_cst_rnd=on  syn_cst_st=-1  synBlockType=primitive  synLatency=0  synBlockId=15
  Constant3 : shlslibv1/Sources/Constant  syn_cst_val=15  syn_cst_format=Specify  syn_cst_wl=4  syn_cst_fl=0  syn_cst_dt=unsigned  syn_cst_rnd=on  syn_cst_st=-1  synBlockType=primitive  synLatency=0  synBlockId=15
  Shifter : shlslibv1/Math Functions/Shifter  syn_shifter_opr=<<  syn_out_f=Automatic  syn_out_wl=16  syn_out_fl=8  syn_out_dt=signed  synBlockType=primitive  synLatency=0  synBlockId=12
  Shifter1 : shlslibv1/Math Functions/Shifter  syn_shifter_opr=>>  syn_out_f=Automatic  syn_out_wl=16  syn_out_fl=8  syn_out_dt=signed  synBlockType=primitive  synLatency=0  synBlockId=12
  Shifter2 : shlslibv1/Math Functions/Shifter  syn_shifter_opr=>>  syn_out_f=Automatic  syn_out_wl=16  syn_out_fl=8  syn_out_dt=signed  synBlockType=primitive  synLatency=0  synBlockId=12
  Shifter3 : shlslibv1/Math Functions/Shifter  syn_shifter_opr=<<  syn_out_f=Automatic  syn_out_wl=16  syn_out_fl=8  syn_out_dt=signed  synBlockType=primitive  synLatency=0  synBlockId=12
  K_iii : Outport
  Kiii1 : Outport  Port=2
  Kiii2 : Outport  Port=3
  Kiii3 : Outport  Port=4
  wires:
  Binary Logic1/1 -> Shifter3/1, Shifter2/1, Binary Logic3/2
  Constant/1 -> Shifter1/2
  Constant1/1 -> Shifter2/2
  Binary Logic2/1 -> Kiii3/1
  Binary Logic4/1 -> Binary Logic2/1
  k_ii/1 -> Binary Logic3/1
  k_ii1/1 -> K_iii/1, Binary Logic1/1
  z/1 -> Binary Logic5/1
  c/1 -> Binary Logic5/2
  k_ii2/1 -> Kiii1/1
  k_ii3/1 -> Shifter/1, Shifter1/1, Kiii2/1
  Binary Logic3/1 -> Binary Logic4/1
  Binary Logic5/1 -> Binary Logic2/2
  Constant2/1 -> Shifter/2
  Shifter1/1 -> Binary Logic6/1
  Shifter/1 -> Binary Logic6/2
  Binary Logic6/1 -> Binary Logic1/2
  Constant3/1 -> Shifter3/2
  Shifter2/1 -> Binary Logic7/1
  Shifter3/1 -> Binary Logic7/2
  Binary Logic7/1 -> Binary Logic4/2

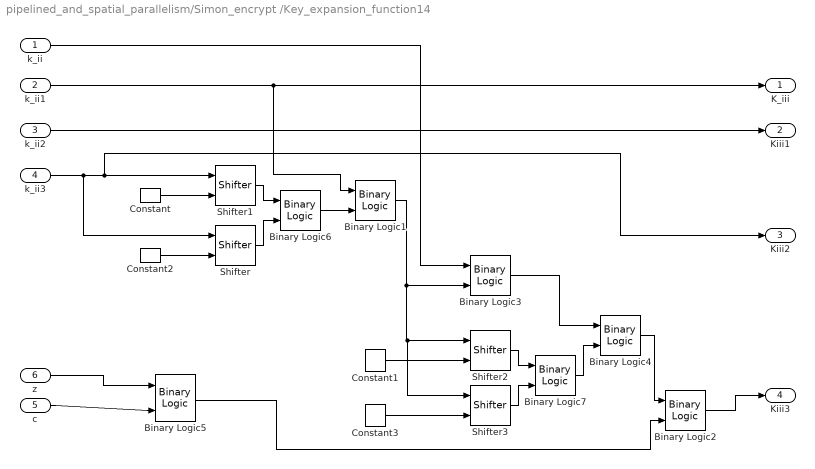
== system pipelined_and_spatial_parallelism/Simon_encrypt /Key_expansion_function14 ==
  k_ii : Inport
  k_ii1 : Inport  Port=2
  k_ii2 : Inport  Port=3
  k_ii3 : Inport  Port=4
  c : Inport  Port=5
  z : Inport  Port=6
  Binary Logic{1..5} (5 alike) : shlslibv1/Math Functions/Binary Logic  syn_binlog_exp=a^b  synBlockType=primitive  synLatency=0  synBlockId=13
  Binary Logic6 : shlslibv1/Math Functions/Binary Logic  syn_binlog_exp=a|b  synBlockType=primitive  synLatency=0  synBlockId=13
  Binary Logic7 : shlslibv1/Math Functions/Binary Logic  syn_binlog_exp=a|b  synBlockType=primitive  synLatency=0  synBlockId=13
  Constant : shlslibv1/Sources/Constant  syn_cst_val=3  syn_cst_format=Specify  syn_cst_wl=4  syn_cst_fl=0  syn_cst_dt=unsigned  syn_cst_rnd=on  syn_cst_st=-1  synBlockType=primitive  synLatency=0  synBlockId=15
  Constant1 : shlslibv1/Sources/Constant  syn_cst_val=1  syn_cst_format=Specify  syn_cst_wl=4  syn_cst_fl=0  syn_cst_dt=unsigned  syn_cst_rnd=on  syn_cst_st=-1  synBlockType=primitive  synLatency=0  synBlockId=15
  Constant2 : shlslibv1/Sources/Constant  syn_cst_val=13  syn_cst_format=Specify  syn_cst_wl=4  syn_cst_fl=0  syn_cst_dt=unsigned  syn_cst_rnd=on  syn_cst_st=-1  synBlockType=primitive  synLatency=0  synBlockId=15
  Constant3 : shlslibv1/Sources/Constant  syn_cst_val=15  syn_cst_format=Specify  syn_cst_wl=4  syn_cst_fl=0  syn_cst_dt=unsigned  syn_cst_rnd=on  syn_cst_st=-1  synBlockType=primitive  synLatency=0  synBlockId=15
  Shifter : shlslibv1/Math Functions/Shifter  syn_shifter_opr=<<  syn_out_f=Automatic  syn_out_wl=16  syn_out_fl=8  syn_out_dt=signed  synBlockType=primitive  synLatency=0  synBlockId=12
  Shifter1 : shlslibv1/Math Functions/Shifter  syn_shifter_opr=>>  syn_out_f=Automatic  syn_out_wl=16  syn_out_fl=8  syn_out_dt=signed  synBlockType=primitive  synLatency=0  synBlockId=12
  Shifter2 : shlslibv1/Math Functions/Shifter  syn_shifter_opr=>>  syn_out_f=Automatic  syn_out_wl=16  syn_out_fl=8  syn_out_dt=signed  synBlockType=primitive  synLatency=0  synBlockId=12
  Shifter3 : shlslibv1/Math Functions/Shifter  syn_shifter_opr=<<  syn_out_f=Automatic  syn_out_wl=16  syn_out_fl=8  syn_out_dt=signed  synBlockType=primitive  synLatency=0  synBlockId=12
  K_iii : Outport
  Kiii1 : Outport  Port=2
  Kiii2 : Outport  Port=3
  Kiii3 : Outport  Port=4
  wires:
  Binary Logic1/1 -> Shifter3/1, Shifter2/1, Binary Logic3/2
  Constant/1 -> Shifter1/2
  Constant1/1 -> Shifter2/2
  Binary Logic2/1 -> Kiii3/1
  Binary Logic4/1 -> Binary Logic2/1
  k_ii/1 -> Binary Logic3/1
  k_ii1/1 -> K_iii/1, Binary Logic1/1
  z/1 -> Binary Logic5/1
  c/1 -> Binary Logic5/2
  k_ii2/1 -> Kiii1/1
  k_ii3/1 -> Shifter/1, Shifter1/1, Kiii2/1
  Binary Logic3/1 -> Binary Logic4/1
  Binary Logic5/1 -> Binary Logic2/2
  Constant2/1 -> Shifter/2
  Shifter1/1 -> Binary Logic6/1
  Shifter/1 -> Binary Logic6/2
  Binary Logic6/1 -> Binary Logic1/2
  Constant3/1 -> Shifter3/2
  Shifter2/1 -> Binary Logic7/1
  Shifter3/1 -> Binary Logic7/2
  Binary Logic7/1 -> Binary Logic4/2

== system pipelined_and_spatial_parallelism/Simon_encrypt /Key_expansion_function15 ==
  k_ii : Inport
  k_ii1 : Inport  Port=2
  k_ii2 : Inport  Port=3
  k_ii3 : Inport  Port=4
  c : Inport  Port=5
  z : Inport  Port=6
  Binary Logic{1..5} (5 alike) : shlslibv1/Math Functions/Binary Logic  syn_binlog_exp=a^b  synBlockType=primitive  synLatency=0  synBlockId=13
  Binary Logic6 : shlslibv1/Math Functions/Binary Logic  syn_binlog_exp=a|b  synBlockType=primitive  synLatency=0  synBlockId=13
  Binary Logic7 : shlslibv1/Math Functions/Binary Logic  syn_binlog_exp=a|b  synBlockType=primitive  synLatency=0  synBlockId=13
  Constant : shlslibv1/Sources/Constant  syn_cst_val=3  syn_cst_format=Specify  syn_cst_wl=4  syn_cst_fl=0  syn_cst_dt=unsigned  syn_cst_rnd=on  syn_cst_st=-1  synBlockType=primitive  synLatency=0  synBlockId=15
  Constant1 : shlslibv1/Sources/Constant  syn_cst_val=1  syn_cst_format=Specify  syn_cst_wl=4  syn_cst_fl=0  syn_cst_dt=unsigned  syn_cst_rnd=on  syn_cst_st=-1  synBlockType=primitive  synLatency=0  synBlockId=15
  Constant2 : shlslibv1/Sources/Constant  syn_cst_val=13  syn_cst_format=Specify  syn_cst_wl=4  syn_cst_fl=0  syn_cst_dt=unsigned  syn_cst_rnd=on  syn_cst_st=-1  synBlockType=primitive  synLatency=0  synBlockId=15
  Constant3 : shlslibv1/Sources/Constant  syn_cst_val=15  syn_cst_format=Specify  syn_cst_wl=4  syn_cst_fl=0  syn_cst_dt=unsigned  syn_cst_rnd=on  syn_cst_st=-1  synBlockType=primitive  synLatency=0  synBlockId=15
  Shifter : shlslibv1/Math Functions/Shifter  syn_shifter_opr=<<  syn_out_f=Automatic  syn_out_wl=16  syn_out_fl=8  syn_out_dt=signed  synBlockType=primitive  synLatency=0  synBlockId=12
  Shifter1 : shlslibv1/Math Functions/Shifter  syn_shifter_opr=>>  syn_out_f=Automatic  syn_out_wl=16  syn_out_fl=8  syn_out_dt=signed  synBlockType=primitive  synLatency=0  synBlockId=12
  Shifter2 : shlslibv1/Math Functions/Shifter  syn_shifter_opr=>>  syn_out_f=Automatic  syn_out_wl=16  syn_out_fl=8  syn_out_dt=signed  synBlockType=primitive  synLatency=0  synBlockId=12
  Shifter3 : shlslibv1/Math Functions/Shifter  syn_shifter_opr=<<  syn_out_f=Automatic  syn_out_wl=16  syn_out_fl=8  syn_out_dt=signed  synBlockType=primitive  synLatency=0  synBlockId=12
  K_iii : Outport
  Kiii1 : Outport  Port=2
  Kiii2 : Outport  Port=3
  Kiii3 : Outport  Port=4
  wires:
  Binary Logic1/1 -> Shifter3/1, Shifter2/1, Binary Logic3/2
  Constant/1 -> Shifter1/2
  Constant1/1 -> Shifter2/2
  Binary Logic2/1 -> Kiii3/1
  Binary Logic4/1 -> Binary Logic2/1
  k_ii/1 -> Binary Logic3/1
  k_ii1/1 -> K_iii/1, Binary Logic1/1
  z/1 -> Binary Logic5/1
  c/1 -> Binary Logic5/2
  k_ii2/1 -> Kiii1/1
  k_ii3/1 -> Shifter/1, Shifter1/1, Kiii2/1
  Binary Logic3/1 -> Binary Logic4/1
  Binary Logic5/1 -> Binary Logic2/2
  Constant2/1 -> Shifter/2
  Shifter1/1 -> Binary Logic6/1
  Shifter/1 -> Binary Logic6/2
  Binary Logic6/1 -> Binary Logic1/2
  Constant3/1 -> Shifter3/2
  Shifter2/1 -> Binary Logic7/1
  Shifter3/1 -> Binary Logic7/2
  Binary Logic7/1 -> Binary Logic4/2
